simulink model "Dual_UKF"  (R2016b)
settings: Solver=FixedStepAuto  StartTime=0.0  StopTime=15  FixedStep=0.00001  MinStep=0.0001  RelTol=1e-3
values from neighbouring files (symbols this model uses):
  Ac = (pi*d^2)/4    (= 2.82743338823e-07)    [SMA_wire_modelling.m]    (also in ut_obs_transform.m; ut_transform.m; ut_transform_obs_param.m)
  As = 68    [Phase_Transformation_Model.m]    (also in SMA_wire_modelling.m = 0.000471238898038; ut_transform.m = 0.000471238898038; ut_transform_param.m = 0.000471238898038)
  Cp = 840    [SMA_wire_modelling.m]    (also in ut_transform.m; ut_transform_param.m)
  D = (Da+Dm)/2    (= 51500000000)    [SMA_wire_modelling.m]    (also in ut_transform.m)
  disp_i = 0.02    [SMA_wire_modelling.m]    (also in ut_obs_transform.m; ut_transform_obs_param.m)
  eps_i = disp_i/L0    (= 0.08)    [SMA_wire_modelling.m]    (also in ut_obs_transform.m; ut_transform_obs_param.m)
  eps_l = 0.067    [SMA_wire_modelling.m]    (also in ut_transform.m)
  h0 = 120    [SMA_wire_modelling.m]    (also in ut_transform.m; ut_transform_param.m)
  h2 = 0.001    [SMA_wire_modelling.m]    (also in ut_transform.m)
  Ks = 100    [SMA_wire_modelling.m]    (also in ut_obs_transform.m = real(qp_km); ut_transform.m = qp_km)
  L0 = 0.25    [SMA_wire_modelling.m]    (also in ut_obs_transform.m; ut_transform.m; ut_transform_obs_param.m; ut_transform_param.m)
  m = 1.14e-4    (= 0.000114)    [SMA_wire_modelling.m]    (also in ut_transform.m; ut_transform_param.m)
  Pp_km_in = eye(2)    [SMA_wire_modelling.m]
  Pqp_km_in = eye(1)    [SMA_wire_modelling.m]
  qp_km_in = Ks_in    (= 99)    [SMA_wire_modelling.m]
  R = 0.8491    [SMA_wire_modelling.m]
  rho_a = 8.37e-7    (= 8.37e-07)    [SMA_wire_modelling.m]    (also in ut_obs_transform.m; ut_transform_obs_param.m)
  rho_m = 9.603e-7    (= 9.603e-07)    [SMA_wire_modelling.m]    (also in ut_obs_transform.m; ut_transform_obs_param.m)
  T_amb = 20    [SMA_wire_modelling.m]    (also in ut_transform.m; ut_transform_param.m)
  theta_T = 550000    [SMA_wire_modelling.m]    (also in ut_transform.m)
  X_dot_km_in = [0 0 0 0 0;0 0 0 0 0]    [SMA_wire_modelling.m]
  xp_km_in = [20;7.0736e6]    [SMA_wire_modelling.m]
  zeta0 = 1    [SMA_wire_modelling.m]    (also in zeta_dot.m)
settings Model: Creator=DAIKI  LastModifiedBy=DAIKI
settings SolverCC: InitialStep=0.0001  AlgebraicLoopSolver=LineSearch
settings DebuggingCC: AlgebraicLoopMsg=none

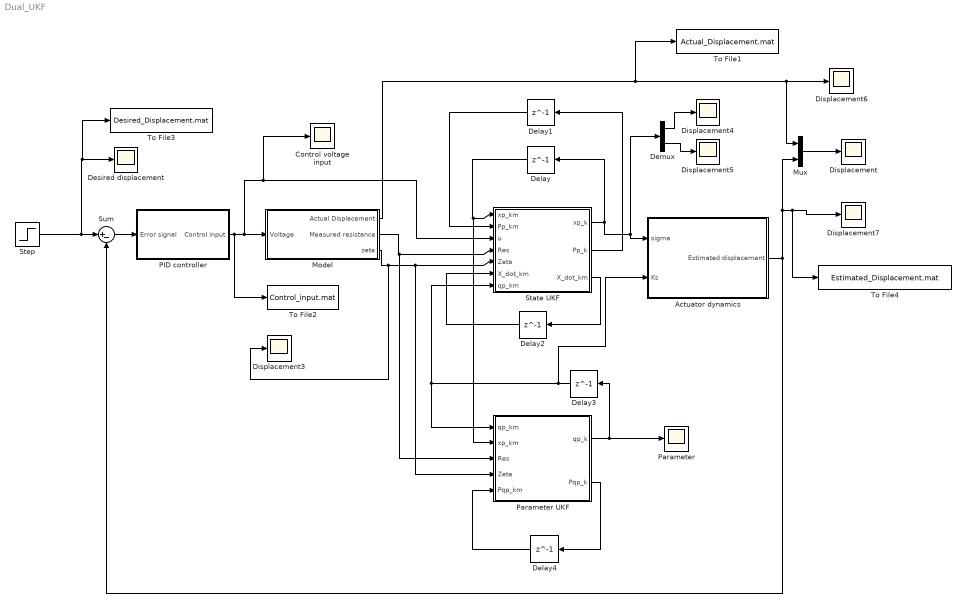
== system Dual_UKF ==
  Actuator dynamics : Subsystem
  Control voltage input : Scope
  Delay : Delay  DelayLength=1  InitialCondition=real(xp_km_in)
  Delay1 : Delay  DelayLength=1  InitialCondition=real(Pp_km_in)
  Delay2 : Delay  DelayLength=1  InitialCondition=real(X_dot_km_in)
  Delay3 : Delay  DelayLength=1  InitialCondition=real(qp_km_in)
  Delay4 : Delay  DelayLength=1  InitialCondition=real(Pqp_km_in)
  Demux : Demux  Outputs=2
  Desired displacement : Scope
  Displacement{,3..7} (6 alike) : Scope
  Model : Subsystem
  Mux : Mux  Inputs=2
  PID controller : Subsystem
  Parameter : Scope
  Parameter UKF : MATLAB Function  TreatAsAtomicUnit=on
  State UKF : MATLAB Function  TreatAsAtomicUnit=on
  Step : Step  Time=0  After=0.025
  Sum : Sum  Inputs=|+-
  To File1 : ToFile  Filename=Actual_Displacement.mat  MatrixName=Dis_act  SaveFormat=Timeseries
  To File2 : ToFile  Filename=Control_input.mat  MatrixName=u_control  SaveFormat=Timeseries
  To File3 : ToFile  Filename=Desired_Displacement.mat  MatrixName=Dis_des  SaveFormat=Timeseries
  To File4 : ToFile  Filename=Estimated_Displacement.mat  MatrixName=Dis_est  SaveFormat=Timeseries
  wires:
  Model/1(Actual Displacement) -> To File1/1, Displacement6/1, Mux/1
  Actuator dynamics/1(Estimated displacement) -> To File4/1, Displacement7/1, Mux/2, Sum/2
  Mux/1 -> Displacement/1
  Step/1 -> To File3/1, Desired displacement/1, Sum/1
  Sum/1 -> PID controller/1(Error signal)
  PID controller/1(Control input) -> To File2/1, Model/1(Voltage), Control voltage input/1, State UKF/3(u)
  State UKF/1(xp_k) -> Delay/1, Demux/1, Actuator dynamics/1(sigma)
  Delay/1 -> Parameter UKF/2(xp_km), State UKF/1(xp_km)
  Delay1/1 -> State UKF/2(Pp_km)
  Model/3(zeta) -> Displacement3/1, Parameter UKF/4(Zeta), State UKF/5(Zeta)
  Model/2(Measured resistance) -> Parameter UKF/3(Res), State UKF/4(Res)
  State UKF/2(Pp_k) -> Delay1/1
  State UKF/3(X_dot_km) -> Delay2/1
  Delay2/1 -> State UKF/6("X_dot_km ")
  Demux/2 -> Displacement5/1
  Demux/1 -> Displacement4/1
  Parameter UKF/1(qp_k) -> Parameter/1, Delay3/1
  Delay3/1 -> Actuator dynamics/2(Ks), State UKF/7(qp_km), Parameter UKF/1(qp_km)
  Parameter UKF/2(Pqp_k) -> Delay4/1
  Delay4/1 -> Parameter UKF/5(Pqp_km)

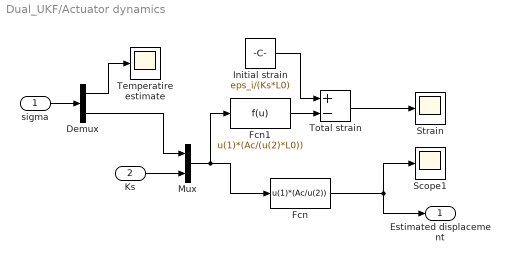
== system Dual_UKF/Actuator dynamics ==
  sigma : Inport
  Ks : Inport  Port=2
  Demux : Demux  Outputs=2
  Fcn : Fcn  Expr=u(1)*(Ac/u(2))
  Fcn1 : Fcn  Expr=u(1)*(Ac/(u(2)*L0))
  Initial strain : Constant  Value=eps_i/(Ks*L0)
  Mux : Mux  Inputs=2
  Scope1 : Scope
  Strain : Scope
  Temperatire estimate : Scope
  Total strain : Sum  Inputs=+-
  Estimated displacement : Outport
  wires:
  Initial strain/1 -> Total strain/1
  Total strain/1 -> Strain/1
  Fcn/1 -> Scope1/1, Estimated displacement/1
  sigma/1 -> Demux/1
  Demux/2 -> Mux/1
  Demux/1 -> Temperatire estimate/1
  Mux/1 -> Fcn1/1, Fcn/1
  Ks/1 -> Mux/2
  Fcn1/1 -> Total strain/2

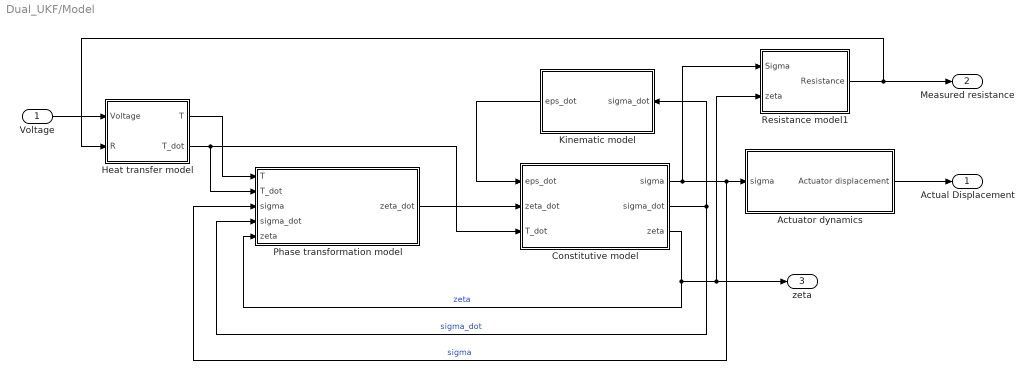
== system Dual_UKF/Model ==
  Voltage : Inport
  Actuator dynamics : Subsystem
  Constitutive model : Subsystem
  Heat transfer model : Subsystem
  Kinematic model : Subsystem
  Phase transformation model : Subsystem
  Resistance model1 : Subsystem
  Actual Displacement : Outport
  Measured resistance : Outport  Port=2
  zeta : Outport  Port=3
  wires:
  Resistance model1/1(Resistance) -> Measured resistance/1, Heat transfer model/2(R)
  Constitutive model/3(zeta) -> zeta/1, Resistance model1/2(zeta), Phase transformation model/5(zeta)  "zeta"
  Heat transfer model/2(T_dot) -> Constitutive model/3(T_dot), Phase transformation model/2(T_dot)
  Heat transfer model/1(T) -> Phase transformation model/1(T)
  Constitutive model/1(sigma) -> Resistance model1/1(Sigma), Phase transformation model/3(sigma), Actuator dynamics/1(sigma)  "sigma"
  Kinematic model/1(eps_dot) -> Constitutive model/1(eps_dot)
  Phase transformation model/1(zeta_dot) -> Constitutive model/2(zeta_dot)
  Constitutive model/2(sigma_dot) -> Phase transformation model/4(sigma_dot), Kinematic model/1(sigma_dot)  "sigma_dot"
  Voltage/1 -> Heat transfer model/1(Voltage)
  Actuator dynamics/1(Actuator displacement) -> Actual Displacement/1

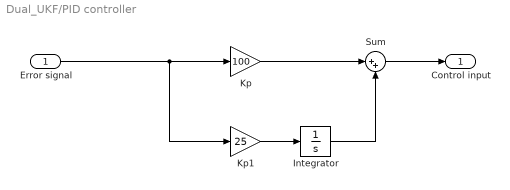
== system Dual_UKF/PID controller ==
  Error signal : Inport
  Integrator : Integrator
  Kp : Gain  Gain=100
  Kp1 : Gain  Gain=25
  Sum : Sum  Inputs=|++
  Control input : Outport
  wires:
  Error signal/1 -> Kp1/1, Kp/1
  Kp/1 -> Sum/1
  Sum/1 -> Control input/1
  Kp1/1 -> Integrator/1
  Integrator/1 -> Sum/2

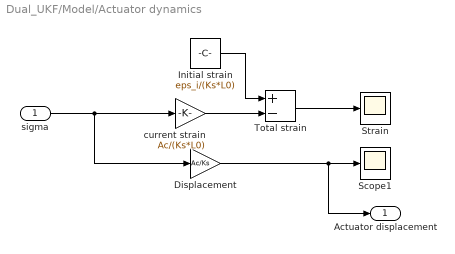
== system Dual_UKF/Model/Actuator dynamics ==
  sigma : Inport
  Displacement : Gain  Gain=Ac/Ks
  Initial strain : Constant  Value=eps_i/(Ks*L0)
  Scope1 : Scope
  Strain : Scope
  Total strain : Sum  Inputs=+-
  current strain : Gain  Gain=Ac/(Ks*L0)
  Actuator displacement : Outport
  wires:
  sigma/1 -> current strain/1, Displacement/1
  Initial strain/1 -> Total strain/1
  current strain/1 -> Total strain/2
  Total strain/1 -> Strain/1
  Displacement/1 -> Actuator displacement/1, Scope1/1

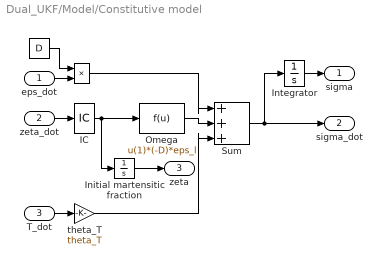
== system Dual_UKF/Model/Constitutive model ==
  eps_dot : Inport
  zeta_dot : Inport  Port=2
  T_dot : Inport  Port=3
  " " : Constant  Value=D
  " " : Product  SaturateOnIntegerOverflow=on  InputSameDT=on  OutDataTypeStr=Inherit: Same as first input
  IC : InitialCondition  Value=0
  Initial martensitic fraction : Integrator  InitialCondition=zeta0  UpperSaturationLimit=1  LowerSaturationLimit=0
  Integrator : Integrator  InitialCondition=(disp_i*Ks)/Ac
  Omega : Fcn  Expr=u(1)*(-D)*eps_l
  Sum : Sum  Inputs=|+|+|+|  SaturateOnIntegerOverflow=on  InputSameDT=on  OutDataTypeStr=Inherit: Same as first input
  theta_T : Gain  Gain=theta_T  SaturateOnIntegerOverflow=on  OutDataTypeStr=Inherit: Same as input  ParamDataTypeStr=Inherit: Same as input
  sigma : Outport
  sigma_dot : Outport  Port=2
  zeta : Outport  Port=3
  wires:
  eps_dot/1 -> " "/2
  " "/1 -> " "/1
  zeta_dot/1 -> IC/1
  T_dot/1 -> theta_T/1
  IC/1 -> Initial martensitic fraction/1, Omega/1
  " "/1 -> Sum/1
  Omega/1 -> Sum/2
  theta_T/1 -> Sum/3
  Sum/1 -> Integrator/1, sigma_dot/1
  Integrator/1 -> sigma/1
  Initial martensitic fraction/1 -> zeta/1

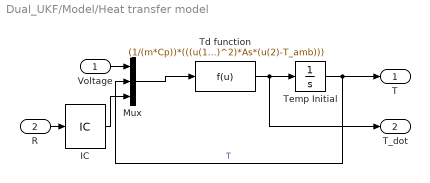
== system Dual_UKF/Model/Heat transfer model ==
  Voltage : Inport
  R : Inport  Port=2
  IC : InitialCondition  Value=R
  Mux : Mux  Inputs=3
  Td function : Fcn  Expr=(1/(m*Cp))*(((u(1)^2)/u(3))-((h0+h2*u(2)^2)*As*(u(2)-T_amb)))
  Temp Initial : Integrator  InitialCondition=T_amb
  T : Outport
  T_dot : Outport  Port=2
  wires:
  Mux/1 -> Td function/1
  Voltage/1 -> Mux/1
  Temp Initial/1 -> T/1, Mux/2  "T"
  Td function/1 -> T_dot/1, Temp Initial/1
  R/1 -> IC/1
  IC/1 -> Mux/3

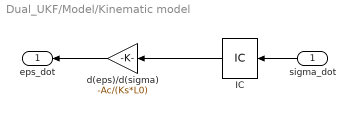
== system Dual_UKF/Model/Kinematic model ==
  sigma_dot : Inport
  IC : InitialCondition  Value=0
  "d(eps)/d(sigma) " : Gain  Gain=-Ac/(Ks*L0)
  eps_dot : Outport
  wires:
  "d(eps)/d(sigma) "/1 -> eps_dot/1
  sigma_dot/1 -> IC/1
  IC/1 -> "d(eps)/d(sigma) "/1

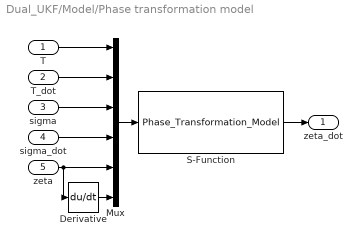
== system Dual_UKF/Model/Phase transformation model ==
  T : Inport
  T_dot : Inport  Port=2
  sigma : Inport  Port=3
  sigma_dot : Inport  Port=4
  zeta : Inport  Port=5
  Derivative : Derivative
  Mux : Mux  Inputs=6
  S-Function : S-Function  FunctionName=Phase_Transformation_Model  SFunctionDeploymentMode=off  EnableBusSupport=off
  zeta_dot : Outport
  wires:
  sigma/1 -> Mux/3
  T_dot/1 -> Mux/2
  T/1 -> Mux/1
  sigma_dot/1 -> Mux/4
  Mux/1 -> S-Function/1
  S-Function/1 -> zeta_dot/1
  Derivative/1 -> Mux/6
  zeta/1 -> Mux/5, Derivative/1

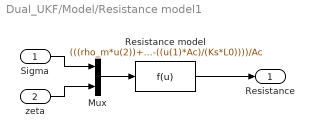
== system Dual_UKF/Model/Resistance model1 ==
  Sigma : Inport
  zeta : Inport  Port=2
  Mux : Mux  Inputs=2
  Resistance model : Fcn  Expr=(((rho_m*u(2))+((1-u(2))*rho_a))*L0*(1+eps_i-((u(1)*Ac)/(Ks*L0))))/Ac
  Resistance : Outport
  wires:
  Resistance model/1 -> Resistance/1
  Mux/1 -> Resistance model/1
  Sigma/1 -> Mux/1
  zeta/1 -> Mux/2

== matlab function Dual_UKF/Parameter UKF ==
  data: qp_km input; qp_k output; Pqp_k output; xp_km input size=[2;1]; Res input; Zeta input; Pqp_km input
function [qp_k,Pqp_k] = UKF_param(qp_km,xp_km,Res,Zeta,Pqp_km)

qp_km = real(qp_km);
xp_km = real(xp_km);
Res = real(Res);
Zeta = real(Zeta);
Pqp_km = real(Pqp_km);

% Model parameters
Num_StateVar = real(2);      %number of state variables
Num_ObsVar = real(1);        %number of observation variables
Num_sigma = real(2*Num_StateVar + 1);      % Number of sigma points
Num_Param = 1;          % number of parameters to be estimated


% Tuning parameters for parameter estimation
alpha_q = 0.01;       % Tuning parameter to define the spread of sigma points
beta_q = 2;           % Tuning parameter for distribution of state (2 is optimal for Gaussian)
kappa_q = 1;          % Tuning parameter for scaling of sigma points (0 or 3- Num_StateVar)             
lambda_q = real(((alpha_q^2)*(Num_StateVar + kappa_q)) - Num_StateVar); % Composite scaling parameter ((alpha^2)*(Num_StateVar + kappa)) - Num_StateVar
gamma_q = real(sqrt(real(Num_StateVar + lambda_q)));       % scaling factor


% Noise
noise_param = 0.00001;
w_param = real(-noise_param + (noise_param - (-noise_param))*rand(1,1));

% Process and Measurement noise characteristics of parameters
Qq = 1e-6;      % 1e-6;
Rq = 5e-7;      % 5e-7;



% Weighting terms for parameters (Num_sigma by 1) or (5 vs 1)
Wm_q = zeros(Num_sigma,1);    % Weights on mean
Wc_q = zeros(Num_sigma,1);    % Weights on covariance

Wm_q(1,1) = real(lambda_q/(Num_StateVar+lambda_q));        % weight for i=0
Wm_q(2:end,1) = real(1/(2*(Num_StateVar+lambda_q)));     % weight for i = 1 to 2*Num_sigma

Wc_q(1,1) = real((lambda_q/(Num_StateVar+lambda_q))+(1 - alpha_q^2 +beta_q)); % weight for i=0 (1 - alpha^2 +beta)
Wc_q(2:end,1) = real(1/(2*(Num_StateVar+lambda_q)));     % weight for 1 = 1 to 2*Num_sigma


qp_km = real(qp_km);
Pqp_km = real(Pqp_km);






%% UKF state estimation

% Calculate sigma point at k-1 time after measurement update
% (2 (Num_StateVar) by 5 (Num_sigma) matrix)
Qm_k = real(sigma_point_param(qp_km,Pqp_km,gamma_q));


%% Time update 


% A priori parameter estimate at k time
% 1 by 1 matrix where row = Num_Param, column = 1
qm_k = real(qp_km + w_param);
Pqm_k = real(Pqp_km + Qq);


% Unscented transform the sigma points using observation function
% (1 by 5) matrix
zeta = real(Zeta);     % phase fraction at k-1 time
Ym_k = real(ut_transform_obs_param(xp_km,Qm_k,Num_ObsVar,Num_sigma,zeta));


% A priori measurement estimate at k time
% 1 by 1 scalar
ym_k = real(timeupdate_obs_param(Wm_q,Ym_k,Num_ObsVar,Num_sigma));


%% Measurement update

% Covariance of the estimated measurement at k time
Pyy_k = real(meaupdate_Pyy_param(Wc_q,Ym_k,ym_k,Rq,Num_sigma,Num_ObsVar));

% Cross covariance between a piori state estimate and measurement
% estimate at k time
Pqy_k = real(meaupdate_Pqy(Wc_q,Qm_k,qm_k,Ym_k,ym_k,Num_sigma,Num_ObsVar,Num_Param));

% Calculate the Kalman gain
K_k = real(Pqy_k/Pyy_k);

% State update after measurement
Res_k = real(Res);               % Actual measurement (taken from open-loop model)
qp_k = real(qm_k + K_k*(Res_k - ym_k));
qp_k = real(qp_k);

% Covariance update after measurement
Pqp_k = Pqm_k - (K_k*Pyy_k*K_k');
Pqp_k = real(Pqp_k);

== matlab function Dual_UKF/State UKF ==
  data: xp_k output size=[2;1]; Pp_k output size=[2;2]; xp_km input; X_dot_km output; Pp_km input; u input; Res input; Zeta input; X_dot_km input size=[2;5]; qp_km input
function [xp_k,Pp_k,X_dot_km] = UKF_state(xp_km,Pp_km,u,Res,Zeta,X_dot_km,qp_km)

u = real(u);
Res = real(Res);
Zeta = real(Zeta);
X_dot_km = real(X_dot_km);
qp_km = real(qp_km);

% Model parameters
Num_StateVar = real(2);      %number of state variables
Num_ObsVar = real(1);        %number of observation variables
Num_sigma = real(2*Num_StateVar + 1);      % Number of sigma points = 

t_sample = real(1e-5);


% Tuning parameters
alpha = real(0.01);       % Tuning parameter to define the spread of sigma points
beta = real(2);           % Tuning parameter for distribution of state (2 is optimal for Gaussian)
kappa = real(1);          % Tuning parameter for scaling of sigma points (0 or 3- Num_StateVar)             
lambda = real(((alpha^2)*(Num_StateVar + kappa)) - Num_StateVar); % Composite scaling parameter ((alpha^2)*(Num_StateVar + kappa)) - Num_StateVar
gamma = real(sqrt(real(Num_StateVar + lambda)));       % scaling factor


% Process and Measurement noise characteristics
w1 = real(1e-10);
w2 = real(1000);
Qv = real([w1*w1 0;0 w2*w2]);  % covariance of process noise (from UKF Gurung [14])
Rv = 0;        % covariance of measurement noise (from UKF Gurung [14])


% Weighting terms (Num_sigma by 1) or (5 vs 1)
Wm = zeros(Num_sigma,1);    % Weights on mean
Wc = zeros(Num_sigma,1);    % Weights on covariance

Wm(1,1) = real(lambda/(Num_StateVar+lambda));        % weight for i=0
Wm(2:end,1) = real(1/(2*(Num_StateVar+lambda)));     % weight for i = 1 to 2*Num_sigma

Wc(1,1) = real((lambda/(Num_StateVar+lambda))+(1 - alpha^2 +beta)); % weight for i=0 (1 - alpha^2 +beta)
Wc(2:end,1) = real(1/(2*(Num_StateVar+lambda)));     % weight for 1 = 1 to 2*Num_sigma

xp_km = real(xp_km);
Pp_km = real(Pp_km);


%% UKF state estimation

% Calculate sigma point at k-1 time after measurement update
% (2 (Num_StateVar) by 5 (Num_sigma) matrix)
Xp_km = real(sigma_point(xp_km,Pp_km,gamma));


%% Time update 

% Unscented transform the sigma at k time before measurement update
% (2 (Num_StateVar) by 5 (Num_sigma) matrix)
u_km = u;                % voltage input at k-1 time
Res_km = Res;               % Actual measurement (taken from open-loop model)
[Xm_k,X_dot_km] = ut_transform(Xp_km,u_km,t_sample,Res_km,X_dot_km,Num_sigma,qp_km);
X_dot_km = real(X_dot_km);

% A priori state estimate at k time
% 2 by 1 matrix where row1 = temp and row 2 = stress
xm_k = real(timeupdate_state(Wm,Xm_k,Num_StateVar,Num_sigma));

% A priori error covariance estimate at k time (2 by 2 matrix)
Pm_k = real(timeupdate_cov(Wc,Xm_k,xm_k,Qv,Num_sigma,Num_StateVar));


% Unscented transform the sigma points using observation function
% (1 by 5) matrix
zeta = real(Zeta);     % phase fraction at k-1 time
Ym_k = real(ut_obs_transform(Xm_k,zeta,Num_ObsVar,qp_km));


% A priori measurement estimate at k time
% 1 by 1 scalar
ym_k = real(timeupdate_obs(Wm,Ym_k,Num_ObsVar,Num_sigma));


%% Measurement update

% Covariance of the estimated measurement at k time
Pyy_k = real(meaupdate_Pyy(Wc,Ym_k,ym_k,Rv,Num_sigma,Num_ObsVar));

% Cross covariance between a piori state estimate and measurement
% estimate at k time
Pxy_k = real(meaupdate_Pxy(Wc,Xm_k,xm_k,Ym_k,ym_k,Num_sigma,Num_ObsVar,Num_StateVar));

% Calculate the Kalman gain
K_k = real(Pxy_k/Pyy_k);

% State update after measurement
Res_k = Res;               % Actual measurement (taken from open-loop model)
xp_k = real(xm_k + K_k*(Res_k - ym_k));
xp_k = real(xp_k);

% Covariance update after measurement
Pp_k = real(Pm_k - (K_k*Pyy_k*K_k'));
Pp_k = real(Pp_k);
